simulink model "conv_inv"  (R2016a)
settings: Solver=VariableStepAuto  StartTime=0.0  StopTime=.3  RelTol=1e-3
libraries: powerlib x28, re_lib x1
settings Model: Creator=Emdadul Haq  LastModifiedBy=Emdadul Haq

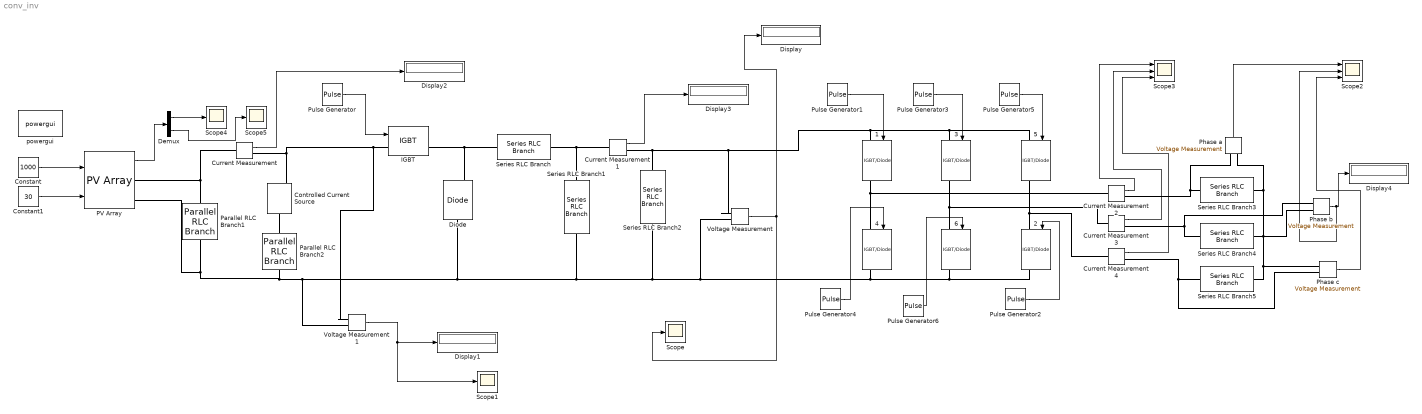
== system conv_inv ==
  {1..6} (6 alike) : powerlib/Power Electronics/IGBT//Diode  Ron=1e-3  Rs=1e5  Cs=inf  Measurements=on
  Constant : Constant  Value=1000  SampleTime=30
  Constant1 : Constant  Value=30
  Controlled Current Source : powerlib/Electrical Sources/Controlled Current Source  Initialize=on  Source_Type=DC  Amplitude=0  Phase=0  Frequency=0  Measurements=Current
  Current Measurement{,1..4} (5 alike) : powerlib/Measurements/Current Measurement  PhasorSimulation=off  OutputType=Complex  PSBequivalent=0
  Demux : Demux  Outputs=2
  Diode : powerlib/Power Electronics/Diode  Ron=0.001  Lon=0  Vf=0.8  IC=0  UseSnubber=off  Rs=500  Cs=250e-9  Measurements=on
  Display{,1..4} (5 alike) : Display
  IGBT : powerlib/Power Electronics/IGBT  Ron=0.001  Lon=0  Vf=1  Tf=1e-6  Tt=2e-6  IC=0  Rs=1e5  Cs=inf  Measurements=on
  PV Array : re_lib/Solar/PV Array  Npar=10  Nser=1  PlotType=array @ 1000 W/m2 & specified temperatures  S_vec="[ 1000  500  100 ]"  Temp_C_vec="[ 45 25  ]"  ModuleName=1Soltech 1STH-215-P  PlotWhenSelected=off  Pm=213.15  Ncell=60  Voc=36.3  Isc=7.84  Vm=29  Im=7.35  beta_Voc_pc=-0.36099  alpha_Isc_pc=0.102  beta_Voc=-0.13104  alpha_Isc=0.007997  IL=7.8649  I0=2.9259e-10  nI=0.98117  Rsh=313.3991  Rs=0.39383  BAL=off  Tc=1e-6  Tfilter=5e-5
  Parallel RLC Branch1 : powerlib/Elements/Parallel RLC Branch  LConnTagsString=a  RConnTagsString=__new0  BranchType=C  Resistance=1  Inductance=1e-3  SetiL0=off  InitialCurrent=0  Capacitance=1000e-6  Setx0=off  InitialVoltage=0  Measurements=None
  Parallel RLC Branch2 : powerlib/Elements/Parallel RLC Branch  LConnTagsString=a  RConnTagsString=__new0  BranchType=R  Resistance=.0255  Inductance=1e-3  SetiL0=off  InitialCurrent=0  Capacitance=470e-6  Setx0=off  InitialVoltage=0  Measurements=None
  Phase a : powerlib/Measurements/Voltage Measurement  PhasorSimulation=off  OutputType=Complex  PSBequivalent=0
  "Phase b " : powerlib/Measurements/Voltage Measurement  PhasorSimulation=off  OutputType=Complex  PSBequivalent=0
  Phase c : powerlib/Measurements/Voltage Measurement  PhasorSimulation=off  OutputType=Complex  PSBequivalent=0
  Pulse Generator : DiscretePulseGenerator  PulseType=Time based  Period=1/10000  PulseWidth=50
  Pulse Generator1 : DiscretePulseGenerator  PulseType=Time based  Period=2e-2  PulseWidth=50
  Pulse Generator2 : DiscretePulseGenerator  PulseType=Time based  Period=2e-2  PulseWidth=50  PhaseDelay=2e-2*(60/360)
  Pulse Generator3 : DiscretePulseGenerator  PulseType=Time based  Period=2e-2  PulseWidth=50  PhaseDelay=2e-2*(120/360)
  Pulse Generator4 : DiscretePulseGenerator  PulseType=Time based  Period=2e-2  PulseWidth=50  PhaseDelay=2e-2*(180/360)
  Pulse Generator5 : DiscretePulseGenerator  PulseType=Time based  Period=2e-2  PulseWidth=50  PhaseDelay=2e-2*(240/360)
  Pulse Generator6 : DiscretePulseGenerator  PulseType=Time based  Period=2e-2  PulseWidth=50  PhaseDelay=2e-2*(300/360)
  Scope{,1,4..5} (4 alike) : Scope
  Scope2 : Scope  NumInputPorts=3
  Scope3 : Scope  NumInputPorts=3
  Series RLC Branch : powerlib/Elements/Series RLC Branch  LConnTagsString=__new0  RConnTagsString=__new0  BranchType=L  Resistance=1  Inductance=1e-3  SetiL0=off  InitialCurrent=0  Capacitance=1e-6  Setx0=off  InitialVoltage=0  Measurements=None
  Series RLC Branch1 : powerlib/Elements/Series RLC Branch  LConnTagsString=__new0  RConnTagsString=__new0  BranchType=C  Resistance=1  Inductance=1e-3  SetiL0=off  InitialCurrent=0  Capacitance=220e-6  Setx0=off  InitialVoltage=0  Measurements=None
  Series RLC Branch2 : powerlib/Elements/Series RLC Branch  LConnTagsString=__new0  RConnTagsString=__new0  BranchType=R  Resistance=10  Inductance=1e-3  SetiL0=off  InitialCurrent=0  Capacitance=1e-6  Setx0=off  InitialVoltage=0  Measurements=None
  Series RLC Branch3 : powerlib/Elements/Series RLC Branch  LConnTagsString=__new0  RConnTagsString=__new0  BranchType=R  Resistance=50  Inductance=1e-3  SetiL0=off  InitialCurrent=0  Capacitance=1e-6  Setx0=off  InitialVoltage=0  Measurements=None
  Series RLC Branch4 : powerlib/Elements/Series RLC Branch  LConnTagsString=__new0  RConnTagsString=__new0  BranchType=R  Resistance=50  Inductance=1e-3  SetiL0=off  InitialCurrent=0  Capacitance=1e-6  Setx0=off  InitialVoltage=0  Measurements=None
  Series RLC Branch5 : powerlib/Elements/Series RLC Branch  LConnTagsString=__new0  RConnTagsString=__new0  BranchType=R  Resistance=50  Inductance=1e-3  SetiL0=off  InitialCurrent=0  Capacitance=1e-6  Setx0=off  InitialVoltage=0  Measurements=None
  Voltage Measurement : powerlib/Measurements/Voltage Measurement  PhasorSimulation=off  OutputType=Complex  PSBequivalent=0
  Voltage Measurement1 : powerlib/Measurements/Voltage Measurement  PhasorSimulation=off  OutputType=Complex  PSBequivalent=0
  powergui : powerlib/powergui  Priority=1  SimulationMode=Continuous  SolverType=Tustin/Backward Euler (TBE)  SampleTime=50e-6  frequency=60  SPID=off  DisableSnubberDevices=off  DisableRonSwitches=off  DisableVfSwitches=off  SwTol=0  DisplayEquations=off  Interpol=off  ExternalGateDelay=off  methode=off  Ts=10  FunctionMessages=off  echomessages=off  HookPort=off  EnableUseOfTLC=off  x0status=blocks  frequencyindice=0  Pbase=100e6  ErrMax=1e-4  Iterations=50  UnitsV=kV  UnitsW=MW  buscounter=0  RestoreLinks=warning  ResistiveCurrentMeasurement=off  Frange=[0:2:500]  Ylog=off  Xlog=on  ShowGrid=off  save=off  variable=ZData  structure=voltage  ZoomFFT=on  StartTime=0.05  cycles=1  DisplayStyle=1  fundamental=50  FreqAxis=off  MaxFrequency=1000  frequencyindicesteady=1  RmsSteady=1  display=off
  wires:
  Constant/1 -> PV Array/1
  Constant1/1 -> PV Array/2
  PV Array/1 -> Demux/1
  Demux/1 -> Scope4/1
  Demux/2 -> Scope5/1
  Pulse Generator/1 -> IGBT/1
  Voltage Measurement/1 -> Scope/1, Display/1
  Voltage Measurement1/1 -> Scope1/1, Display1/1
  Current Measurement/1 -> Display2/1
  Current Measurement1/1 -> Display3/1
  Pulse Generator1/1 -> 1/1
  Pulse Generator2/1 -> 2/1
  Pulse Generator3/1 -> 3/1
  Pulse Generator4/1 -> 4/1
  Pulse Generator5/1 -> 5/1
  Pulse Generator6/1 -> 6/1
  Phase a/1 -> Scope2/1
  "Phase b "/1 -> Scope2/2, Display4/1
  Phase c/1 -> Scope2/3
  Current Measurement2/1 -> Scope3/1
  Current Measurement3/1 -> Scope3/2
  Current Measurement4/1 -> Scope3/3
  connections:
  6/RConn1 -- Series RLC Branch2/LConn1 -- Series RLC Branch1/RConn1 -- Voltage Measurement1/LConn2 -- PV Array/RConn2 -- Parallel RLC Branch1/RConn1 -- Parallel RLC Branch2/RConn1 -- Diode/LConn1 -- Voltage Measurement/LConn2 -- 4/RConn1 -- 2/RConn1
  Parallel RLC Branch1/LConn1 -- PV Array/RConn1 -- Current Measurement/LConn1
  Controlled Current Source/LConn1 -- Voltage Measurement1/LConn1 -- IGBT/LConn1 -- Current Measurement/RConn1
  Controlled Current Source/RConn1 -- Parallel RLC Branch2/LConn1
  Series RLC Branch/LConn1 -- Diode/RConn1 -- IGBT/RConn1
  Series RLC Branch/RConn1 -- Current Measurement1/LConn1 -- Series RLC Branch1/LConn1
  3/LConn1 -- Voltage Measurement/LConn1 -- Series RLC Branch2/RConn1 -- Current Measurement1/RConn1 -- 1/LConn1 -- 5/LConn1
  1/RConn1 -- Current Measurement2/LConn1 -- 4/LConn1
  3/RConn1 -- Current Measurement3/LConn1 -- 6/LConn1
  5/RConn1 -- 2/LConn1 -- Current Measurement4/LConn1
  Series RLC Branch3/RConn1 -- Phase c/LConn1 -- Series RLC Branch5/RConn1 -- "Phase b "/LConn2 -- Series RLC Branch4/RConn1 -- Phase a/LConn2
  Series RLC Branch3/LConn1 -- Phase a/LConn1 -- Current Measurement2/RConn1
  "Phase b "/LConn1 -- Series RLC Branch4/LConn1 -- Current Measurement3/RConn1
  Series RLC Branch5/LConn1 -- Current Measurement4/RConn1 -- Phase c/LConn2
